simulink model "homework4_simu"  (R2018b)
settings: Solver=VariableStepAuto  StartTime=0.0  StopTime=10.0  RelTol=1e-3
values from neighbouring files (symbols this model uses):
  gamma = [0.632; 0.368]    [homework4.m]
  K = [1.368 0.2143]    [homework4.m]
  L = [0 1]*inv(W)*P    [homework4.m]
  m = 1/1.263    (= 0.791765637371)    [homework4.m]
  phi = [0.368 0; 0.632 1]    [homework4.m]
settings Model: Creator=Henkka  LastModifiedBy=Henkka

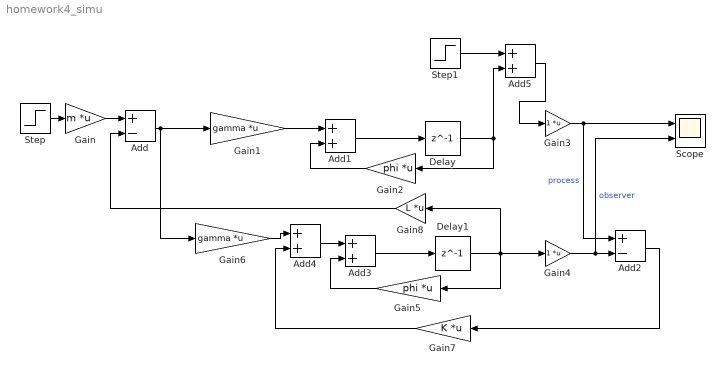
== system homework4_simu ==
  Add : Sum  Inputs=+-
  Add{1,3..5} (4 alike) : Sum
  Add2 : Sum  Inputs=+-
  Delay : Delay  DelayLength=1  InitialCondition=0
  Delay1 : Delay  DelayLength=1  InitialCondition=0
  Gain : Gain  Gain=m  Multiplication=Matrix(K*u)
  Gain1 : Gain  Gain=gamma  Multiplication=Matrix(K*u)
  Gain2 : Gain  Gain=phi  Multiplication=Matrix(K*u)
  Gain3 : Gain  Multiplication=Matrix(K*u)
  Gain4 : Gain  Multiplication=Matrix(K*u)
  Gain5 : Gain  Gain=phi  Multiplication=Matrix(K*u)
  Gain6 : Gain  Gain=gamma  Multiplication=Matrix(K*u)
  Gain7 : Gain  Gain=K  Multiplication=Matrix(K*u)
  Gain8 : Gain  Gain=L  Multiplication=Matrix(K*u)
  Scope : Scope  NumInputPorts=2
  Step : Step  After=10  SampleTime=0
  Step1 : Step  After=0.1  SampleTime=0
  wires:
  Gain/1 -> Add/1
  Add/1 -> Gain6/1, Gain1/1
  Gain1/1 -> Add1/1
  Gain2/1 -> Add1/2
  Add1/1 -> Delay/1
  Delay/1 -> Gain2/1, Add5/2
  Gain4/1 -> Scope/2, Add2/2  "observer"
  Delay1/1 -> Gain8/1, Gain5/1, Gain4/1
  Add3/1 -> Delay1/1
  Gain5/1 -> Add3/2
  Add4/1 -> Add3/1
  Gain6/1 -> Add4/1
  Add2/1 -> Gain7/1
  Gain8/1 -> Add/2
  Step/1 -> Gain/1
  Gain7/1 -> Add4/2
  Step1/1 -> Add5/1
  Add5/1 -> Gain3/1
  Gain3/1 -> Add2/1, Scope/1  "process"
